simulink model "travelling_wind"  (R2019b)
settings: Solver=VariableStepAuto  StartTime=0.0  StopTime=10.0  RelTol=1e-3
values from neighbouring files (symbols this model uses):
  wind_amplitude = 1    [create_travelling_wind_rectangle.m]    (also in create_travelling_wind_sine.m; run_wheat_line_sway_experiment.m)
  wind_frequency = 2    [create_travelling_wind_rectangle.m]    (also in create_travelling_wind_sine.m = 5; run_wheat_line_sway_experiment.m = 50)
  wind_phase_cycle = 5    [create_travelling_wind_rectangle.m]    (also in create_travelling_wind_sine.m = 10; run_wheat_line_sway_experiment.m = 250)
settings Model: Creator=yz655  LastModifiedBy=yz655

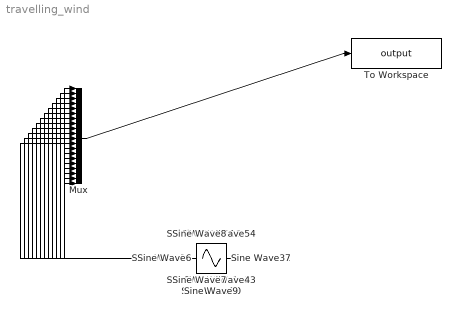
== system travelling_wind ==
  Mux : Mux  Inputs=20
  Sine Wave1 : Sin  Amplitude=wind_amplitude  Frequency=wind_frequency  Phase=2*pi/wind_phase_cycle*1  SampleTime=0
  Sine Wave10 : Sin  Amplitude=wind_amplitude  Frequency=wind_frequency  Phase=2*pi/wind_phase_cycle*10  SampleTime=0
  Sine Wave11 : Sin  Amplitude=wind_amplitude  Frequency=wind_frequency  Phase=2*pi/wind_phase_cycle*11  SampleTime=0
  Sine Wave12 : Sin  Amplitude=wind_amplitude  Frequency=wind_frequency  Phase=2*pi/wind_phase_cycle*12  SampleTime=0
  Sine Wave13 : Sin  Amplitude=wind_amplitude  Frequency=wind_frequency  Phase=2*pi/wind_phase_cycle*13  SampleTime=0
  Sine Wave14 : Sin  Amplitude=wind_amplitude  Frequency=wind_frequency  Phase=2*pi/wind_phase_cycle*14  SampleTime=0
  Sine Wave15 : Sin  Amplitude=wind_amplitude  Frequency=wind_frequency  Phase=2*pi/wind_phase_cycle*15  SampleTime=0
  Sine Wave16 : Sin  Amplitude=wind_amplitude  Frequency=wind_frequency  Phase=2*pi/wind_phase_cycle*16  SampleTime=0
  Sine Wave17 : Sin  Amplitude=wind_amplitude  Frequency=wind_frequency  Phase=2*pi/wind_phase_cycle*17  SampleTime=0
  Sine Wave18 : Sin  Amplitude=wind_amplitude  Frequency=wind_frequency  Phase=2*pi/wind_phase_cycle*18  SampleTime=0
  Sine Wave19 : Sin  Amplitude=wind_amplitude  Frequency=wind_frequency  Phase=2*pi/wind_phase_cycle*19  SampleTime=0
  Sine Wave2 : Sin  Amplitude=wind_amplitude  Frequency=wind_frequency  Phase=2*pi/wind_phase_cycle*2  SampleTime=0
  Sine Wave20 : Sin  Amplitude=wind_amplitude  Frequency=wind_frequency  Phase=2*pi/wind_phase_cycle*20  SampleTime=0
  Sine Wave3 : Sin  Amplitude=wind_amplitude  Frequency=wind_frequency  Phase=2*pi/wind_phase_cycle*3  SampleTime=0
  Sine Wave4 : Sin  Amplitude=wind_amplitude  Frequency=wind_frequency  Phase=2*pi/wind_phase_cycle*4  SampleTime=0
  Sine Wave5 : Sin  Amplitude=wind_amplitude  Frequency=wind_frequency  Phase=2*pi/wind_phase_cycle*5  SampleTime=0
  Sine Wave6 : Sin  Amplitude=wind_amplitude  Frequency=wind_frequency  Phase=2*pi/wind_phase_cycle*6  SampleTime=0
  Sine Wave7 : Sin  Amplitude=wind_amplitude  Frequency=wind_frequency  Phase=2*pi/wind_phase_cycle*7  SampleTime=0
  Sine Wave8 : Sin  Amplitude=wind_amplitude  Frequency=wind_frequency  Phase=2*pi/wind_phase_cycle*8  SampleTime=0
  Sine Wave9 : Sin  Amplitude=wind_amplitude  Frequency=wind_frequency  Phase=2*pi/wind_phase_cycle*9  SampleTime=0
  To Workspace : ToWorkspace  VariableName=output  SaveFormat=Timeseries  SampleTime=-1
  wires:
  Sine Wave1/1 -> Mux/1
  Sine Wave2/1 -> Mux/2
  Sine Wave3/1 -> Mux/3
  Sine Wave4/1 -> Mux/4
  Sine Wave5/1 -> Mux/5
  Sine Wave6/1 -> Mux/6
  Sine Wave7/1 -> Mux/7
  Sine Wave8/1 -> Mux/8
  Sine Wave9/1 -> Mux/9
  Sine Wave10/1 -> Mux/10
  Sine Wave11/1 -> Mux/11
  Sine Wave12/1 -> Mux/12
  Sine Wave13/1 -> Mux/13
  Sine Wave14/1 -> Mux/14
  Sine Wave15/1 -> Mux/15
  Sine Wave16/1 -> Mux/16
  Sine Wave17/1 -> Mux/17
  Sine Wave18/1 -> Mux/18
  Sine Wave19/1 -> Mux/19
  Sine Wave20/1 -> Mux/20
  Mux/1 -> To Workspace/1
